simulink model "dbx_control"  (R2015a)
settings: Solver=FixedStepDiscrete  SolverMode=SingleTasking  StartTime=0.0  StopTime=20  FixedStep=T_ctrl  RelTol=1e-3
undefined symbols (not defined in the file): A_l_max_x, A_M, A_z_max, CG, epsilon, Flaps_ang_deg, g, Hover_eta_23, Hover_throtle_1, Hover_throtle_23, I_BAC, L_M, m, PID_phi_dot_Kd, PID_phi_dot_Ki, PID_phi_dot_Kp, PID_phi_Kd, PID_phi_Ki, PID_phi_Kp, PID_theta_dot_Kd, PID_theta_dot_Ki, PID_theta_dot_Kp, PID_theta_Kd, PID_theta_Ki, PID_theta_Kp, psi_f_i, psi_K_b, psi_tau, Roll_pich_sens, Servo_calib, T_ctrl, Throtle_sens, v_i0, Yaw_sens
libraries: DBX_model x29, DBX_Control_lib x15, simulink x7, DBX_Control x3
(part 1 of 2)
settings Model: ExtModeTrigDuration=5000  TunableVars=Flaps_ang_deg,PID_phi_Kd,PID_phi_Ki,PID_phi_Kp,PID_phi_dot_Kd,PID_phi_dot_Ki,PID_phi_dot_Kp,PID_theta_Kd,PID_theta_Ki,PID_theta_Kp,PID_theta_dot_Kd,PID_theta_dot_Ki,PID_theta_dot_Kp,Roll_pich_sens,Throtle_sens,Yaw_sens,p_K_b,p_tau,phi_K_b,phi_f_i,phi_tau,psi_K_b,psi_f_i,psi_tau,q_K_b,q_tau,r_K_b,r_tau,theta_K_b,theta_f_i,theta_tau  TunableVarsStorageClass=Auto,Auto,Auto,Auto,Auto,Auto,Auto,Auto,Auto,Auto,Auto,Auto,Auto,Auto,Auto,Auto,Auto,Auto,Auto,Auto,Auto,Auto,Auto,Auto,Auto,Auto,Auto,Auto,Auto,Auto,Auto  TunableVarsTypeQualifier=,,,,,,,,,,,,,,,,,,,,,,,,,,,,,,  Creator=DavidTorres  LastModifiedBy=david
settings DataIOCC: LimitDataPoints=off  SaveOutput=off  SignalLogging=off  DSMLogging=off  VisualizeSimOutput=off  SaveTime=off
settings OptimizationCC: InlineParams=on  UseDivisionForNetSlopeComputation=on  UseFloatMulNetSlope=on  UseSpecifiedMinMax=on  InlineInvariantSignals=on  StrengthReduction=on  ZeroExternalMemoryAtStartup=off  ZeroInternalMemoryAtStartup=off  NoFixptDivByZeroProtection=on  EfficientFloat2IntCast=on  OptimizeModelRefInitCode=on  MaxStackSize=64  SimCompilerOptimization=on
settings DebuggingCC: AlgebraicLoopMsg=error  SaveWithParameterizedLinksMsg=none  IntegerOverflowMsg=error  StrictBusMsg=ErrorOnBusTreatedAsVector  IntegerSaturationMsg=error
settings HardwareCC: ProdLargestAtomicInteger=Long  ProdLargestAtomicFloat=Float  ProdIntDivRoundTo=Zero  ProdEndianess=LittleEndian  ProdHWDeviceType=ARM Compatible->ARM 7  TargetLongLongMode=on  TargetIntDivRoundTo=Zero  TargetEndianess=LittleEndian  TargetHWDeviceType=MATLAB Host  ProdEqTarget=off
settings ModelReferenceCC: ModelReferenceNumInstancesAllowed=Single  ModelReferencePassRootInputsByReference=off
settings RTWCC: SystemTargetFile=ert.tlc  GenCodeOnly=on  TemplateMakefile=ert_default_tmf  Description=Embedded Coder  BuildConfiguration=Faster Runs
settings CodeAppCC: IgnoreCustomStorageClasses=off
settings ERTTargetCC: GenerateSampleERTMain=off  ParMdlRefBuildCompliant=on  CompOptLevelCompliant=on  ConcurrentExecutionCompliant=on  CombineSignalStateStructs=on  SuppressErrorStatus=on  ERTFirstTimeCompliant=on  SupportNonFinite=off  SupportComplex=off  SupportContinuousTime=off  ModelStepFunctionPrototypeControlCompliant=on  CPPClassGenCompliant=on  InlinedParameterPlacement=Hierarchical  ERTCustomFileTemplate=example_file_process.tlc

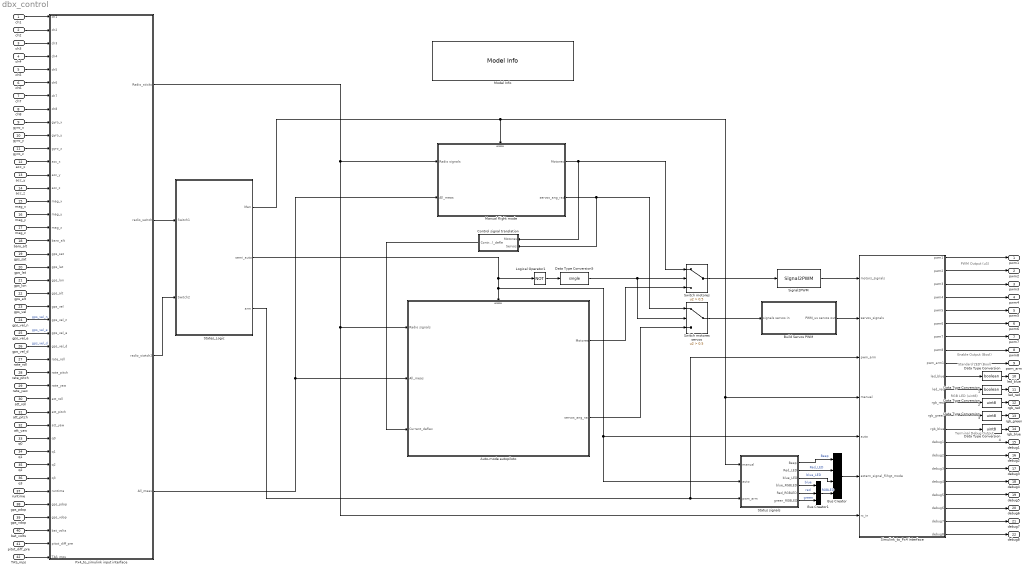
== system dbx_control ==
  note: Terminal Debug Output
  note: RGB LED (uint8)
  note: Standard LED (Bool)
  note: PWM Output (uS)
  note: Enable Output (Bool)
  ch1 : Inport  OutDataTypeStr=double  PortDimensions=[1,1]  SampleTime=T_ctrl
  ch2 : Inport  Port=2  OutDataTypeStr=double  PortDimensions=[1,1]  SampleTime=T_ctrl
  ch3 : Inport  Port=3  OutDataTypeStr=double  PortDimensions=[1,1]  SampleTime=T_ctrl
  ch4 : Inport  Port=4  OutDataTypeStr=double  PortDimensions=[1,1]  SampleTime=T_ctrl
  ch5 : Inport  Port=5  OutDataTypeStr=double  PortDimensions=[1,1]  SampleTime=T_ctrl
  ch6 : Inport  Port=6  OutDataTypeStr=double  PortDimensions=[1,1]  SampleTime=T_ctrl
  ch7 : Inport  Port=7  OutDataTypeStr=double  PortDimensions=[1,1]  SampleTime=T_ctrl
  ch8 : Inport  Port=8  OutDataTypeStr=double  PortDimensions=[1,1]  SampleTime=T_ctrl
  gyro_x : Inport  Port=9  OutDataTypeStr=double  PortDimensions=[1,1]  SampleTime=T_ctrl
  gyro_y : Inport  Port=10  OutDataTypeStr=double  PortDimensions=[1,1]  SampleTime=T_ctrl
  gyro_z : Inport  Port=11  OutDataTypeStr=double  PortDimensions=[1,1]  SampleTime=T_ctrl
  acc_x : Inport  Port=12  OutDataTypeStr=double  PortDimensions=[1,1]  SampleTime=T_ctrl
  acc_y : Inport  Port=13  OutDataTypeStr=double  PortDimensions=[1,1]  SampleTime=T_ctrl
  acc_z : Inport  Port=14  OutDataTypeStr=double  PortDimensions=[1,1]  SampleTime=T_ctrl
  mag_x : Inport  Port=15  OutDataTypeStr=double  PortDimensions=[1,1]  SampleTime=T_ctrl
  mag_y : Inport  Port=16  OutDataTypeStr=double  PortDimensions=[1,1]  SampleTime=T_ctrl
  mag_z : Inport  Port=17  OutDataTypeStr=double  PortDimensions=[1,1]  SampleTime=T_ctrl
  baro_alt : Inport  Port=18  OutDataTypeStr=double  PortDimensions=[1,1]  SampleTime=T_ctrl
  gps_sat : Inport  Port=19  OutDataTypeStr=double  PortDimensions=[1,1]  SampleTime=T_ctrl
  gps_lat : Inport  Port=20  OutDataTypeStr=double  PortDimensions=[1,1]  SampleTime=T_ctrl
  gps_lon : Inport  Port=21  OutDataTypeStr=double  PortDimensions=[1,1]  SampleTime=T_ctrl
  gps_alt : Inport  Port=22  OutDataTypeStr=double  PortDimensions=[1,1]  SampleTime=T_ctrl
  gps_vel : Inport  Port=23  OutDataTypeStr=double  PortDimensions=[1,1]  SampleTime=T_ctrl
  gps_vel_n : Inport  Port=24  OutDataTypeStr=double  PortDimensions=[1,1]  SampleTime=T_ctrl
  gps_vel_e : Inport  Port=25  OutDataTypeStr=double  PortDimensions=[1,1]  SampleTime=T_ctrl
  gps_vel_d : Inport  Port=26  OutDataTypeStr=double  PortDimensions=[1,1]  SampleTime=T_ctrl
  rate_roll : Inport  Port=27  OutDataTypeStr=double  PortDimensions=[1,1]  SampleTime=T_ctrl
  rate_pitch : Inport  Port=28  OutDataTypeStr=double  PortDimensions=[1,1]  SampleTime=T_ctrl
  rate_yaw : Inport  Port=29  OutDataTypeStr=double  PortDimensions=[1,1]  SampleTime=T_ctrl
  att_roll : Inport  Port=30  OutDataTypeStr=double  PortDimensions=[1,1]  SampleTime=T_ctrl
  att_pitch : Inport  Port=31  OutDataTypeStr=double  PortDimensions=[1,1]  SampleTime=T_ctrl
  att_yaw : Inport  Port=32  OutDataTypeStr=double  PortDimensions=[1,1]  SampleTime=T_ctrl
  q0 : Inport  Port=33  OutDataTypeStr=double  PortDimensions=[1,1]  SampleTime=T_ctrl
  q1 : Inport  Port=34  OutDataTypeStr=double  PortDimensions=[1,1]  SampleTime=T_ctrl
  q2 : Inport  Port=35  OutDataTypeStr=double  PortDimensions=[1,1]  SampleTime=T_ctrl
  q3 : Inport  Port=36  OutDataTypeStr=double  PortDimensions=[1,1]  SampleTime=T_ctrl
  runtime : Inport  Port=37  OutDataTypeStr=double  PortDimensions=[1,1]  SampleTime=T_ctrl
  gps_pdop : Inport  Port=38  OutDataTypeStr=double  PortDimensions=[1,1]  SampleTime=T_ctrl
  gps_vdop : Inport  Port=39  OutDataTypeStr=double  PortDimensions=[1,1]  SampleTime=T_ctrl
  bat_volts : Inport  Port=40  OutDataTypeStr=double  PortDimensions=[1,1]  SampleTime=T_ctrl
  pitot_diff_pre : Inport  Port=41  OutDataTypeStr=double  SampleTime=T_ctrl
  TAS_mps : Inport  Port=42  OutDataTypeStr=double  SampleTime=T_ctrl
  Auto-mode autopiloto : Subsystem  TreatAsAtomicUnit=on
  Build Servos PWM : Subsystem  TreatAsAtomicUnit=on
  Bus Creator : BusCreator
  Bus Creator1 : BusCreator  Inputs=3
  Control signal translation : Subsystem  TreatAsAtomicUnit=on
  Data Type Conversion : DataTypeConversion  OutDataTypeStr=boolean
  Data Type Conversion1 : DataTypeConversion  OutDataTypeStr=boolean
  Data Type Conversion2 : DataTypeConversion  OutDataTypeStr=uint8
  Data Type Conversion3 : DataTypeConversion  OutDataTypeStr=uint8
  Data Type Conversion4 : DataTypeConversion  OutDataTypeStr=uint8
  Data Type Conversion5 : DataTypeConversion  OutDataTypeStr=single
  Logical Operator1 : Logic  Operator=NOT  IconShape=distinctive  AllPortsSameDT=off  OutDataTypeStr=boolean
  Manual flight mode : Subsystem  TreatAsAtomicUnit=on
  Model Info : simulink/Model-Wide Utilities/Model Info  Frame=on  DisplayStringWithTags=|  HorizontalTextAlignment=Center  LeftAlignmentValue=0.5  SourceBlockDiagram=dbx_control  TagMaxNumber=20
      | Model Info
      | 
      | Creado por %<Creator>
      | Modificado el %<LastModificationDate> por %<LastModifiedBy>
      | Version %<ModelVersion>
  Px4_to_simulink input interface : Subsystem
  Signal2PWM : DBX_model/Signal2PWM  b=1  d=0  a=DBX_PWM.Motors.Max_PWM  c=DBX_PWM.Motors.Min_PWM
  Simulink_to_Px4 interface : Subsystem
  States_Logic : Subsystem
  Status signals : Subsystem  TreatAsAtomicUnit=on
  Switch motores : Switch  Criteria=u2 > Threshold  Threshold=0.5
  Switch motores servos : Switch  Criteria=u2 > Threshold  Threshold=0.5
  pwm1 : Outport  PortDimensions=[1,1]
  pwm2 : Outport  Port=2  PortDimensions=[1,1]
  pwm3 : Outport  Port=3  PortDimensions=[1,1]
  pwm4 : Outport  Port=4  PortDimensions=[1,1]
  pwm5 : Outport  Port=5  PortDimensions=[1,1]
  pwm6 : Outport  Port=6  PortDimensions=[1,1]
  pwm7 : Outport  Port=7  PortDimensions=[1,1]
  pwm8 : Outport  Port=8  PortDimensions=[1,1]
  pwm_arm : Outport  Port=9  PortDimensions=[1,1]
  led_blue : Outport  Port=10  OutDataTypeStr=boolean  PortDimensions=[1,1]
  led_red : Outport  Port=11  OutDataTypeStr=boolean  PortDimensions=[1,1]
  rgb_red : Outport  Port=12  OutDataTypeStr=uint8  PortDimensions=[1,1]
  rgb_green : Outport  Port=13  OutDataTypeStr=uint8  PortDimensions=[1,1]
  rgb_blue : Outport  Port=14  OutDataTypeStr=uint8  PortDimensions=[1,1]
  debug1 : Outport  Port=15  PortDimensions=[1,1]
  debug2 : Outport  Port=16  PortDimensions=[1,1]
  debug3 : Outport  Port=17  PortDimensions=[1,1]
  debug4 : Outport  Port=18  PortDimensions=[1,1]
  debug5 : Outport  Port=19  PortDimensions=[1,1]
  debug6 : Outport  Port=20  PortDimensions=[1,1]
  debug7 : Outport  Port=21  PortDimensions=[1,1]
  debug8 : Outport  Port=22  PortDimensions=[1,1]
  wires:
  Switch motores/1 -> Signal2PWM/1
  Switch motores servos/1 -> Build Servos PWM/1(signals servos in)
  Status signals/1(Beep) -> Bus Creator/1  "Beep"
  Status signals/2(Red_LED) -> Bus Creator/2  "Red_LED"
  Status signals/3(blue_LED) -> Bus Creator/3  "blue_LED"
  Status signals/4(blue_RGBLED) -> Bus Creator1/1  "blue"
  Status signals/5(Red_RGBLED) -> Bus Creator1/2  "red"
  Status signals/6(green_RGBLED) -> Bus Creator1/3  "green"
  Bus Creator1/1 -> Bus Creator/4  "RGBLED"
  Simulink_to_Px4 interface/1(pwm1) -> pwm1/1
  Simulink_to_Px4 interface/2(pwm2) -> pwm2/1
  Simulink_to_Px4 interface/3(pwm3) -> pwm3/1
  Simulink_to_Px4 interface/4(pwm4) -> pwm4/1
  Simulink_to_Px4 interface/5(pwm5) -> pwm5/1
  Simulink_to_Px4 interface/6(pwm6) -> pwm6/1
  Simulink_to_Px4 interface/7(pwm7) -> pwm7/1
  Simulink_to_Px4 interface/8(pwm8) -> pwm8/1
  Simulink_to_Px4 interface/10(led_blue) -> Data Type Conversion/1
  Simulink_to_Px4 interface/11(led_red) -> Data Type Conversion1/1
  Simulink_to_Px4 interface/15(debug1) -> debug1/1
  Simulink_to_Px4 interface/17(debug3) -> debug3/1
  Simulink_to_Px4 interface/18(debug4) -> debug4/1
  Simulink_to_Px4 interface/9(pwm_arm1) -> pwm_arm/1
  Simulink_to_Px4 interface/12(rgb_red) -> Data Type Conversion2/1
  Simulink_to_Px4 interface/13(rgb_green) -> Data Type Conversion3/1
  Simulink_to_Px4 interface/14(rgb_blue) -> Data Type Conversion4/1
  Simulink_to_Px4 interface/20(debug6) -> debug6/1
  Simulink_to_Px4 interface/21(debug7) -> debug7/1
  Simulink_to_Px4 interface/22(debug8) -> debug8/1
  Simulink_to_Px4 interface/19(debug5) -> debug5/1
  Data Type Conversion/1 -> led_blue/1
  Data Type Conversion1/1 -> led_red/1
  Data Type Conversion2/1 -> rgb_red/1
  Data Type Conversion3/1 -> rgb_green/1
  Data Type Conversion4/1 -> rgb_blue/1
  Simulink_to_Px4 interface/16(debug2) -> debug2/1
  Signal2PWM/1 -> Simulink_to_Px4 interface/1(motors_signals)
  Build Servos PWM/1(PWM_us servos out) -> Simulink_to_Px4 interface/2(servos_signals)
  Bus Creator/1 -> Simulink_to_Px4 interface/6(extern_signal_flihgt_mode)
  Manual flight mode/2(servos_ang_rad) -> Switch motores servos/1, Control signal translation/2(Servos)
  Auto-mode autopiloto/1(Motores) -> Switch motores/3
  Auto-mode autopiloto/2(servos_ang_rad) -> Switch motores servos/3
  Data Type Conversion5/1 -> Switch motores/2, Switch motores servos/2
  Px4_to_simulink input interface/4(All_meas) -> Auto-mode autopiloto/2(All_meas), Manual flight mode/2(All_meas)
  Px4_to_simulink input interface/1(Radio_sticks) -> Manual flight mode/1(Radio signals), Simulink_to_Px4 interface/7(rc_in), Auto-mode autopiloto/1(Radio signals)
  Manual flight mode/1(Motores) -> Switch motores/1, Control signal translation/1(Motores)
  Control signal translation/1(Control_defle) -> Auto-mode autopiloto/3(Current_deflex)
  ch1/1 -> Px4_to_simulink input interface/1(ch1)
  ch2/1 -> Px4_to_simulink input interface/2(ch2)
  ch3/1 -> Px4_to_simulink input interface/3(ch3)
  ch4/1 -> Px4_to_simulink input interface/4(ch4)
  ch5/1 -> Px4_to_simulink input interface/5(ch5)
  ch6/1 -> Px4_to_simulink input interface/6(ch6)
  ch7/1 -> Px4_to_simulink input interface/7(ch7)
  ch8/1 -> Px4_to_simulink input interface/8(ch8)
  gyro_x/1 -> Px4_to_simulink input interface/9(gyro_x)
  gyro_y/1 -> Px4_to_simulink input interface/10(gyro_y)
  gyro_z/1 -> Px4_to_simulink input interface/11(gyro_z)
  acc_x/1 -> Px4_to_simulink input interface/12(acc_x)
  acc_y/1 -> Px4_to_simulink input interface/13(acc_y)
  acc_z/1 -> Px4_to_simulink input interface/14(acc_z)
  mag_z/1 -> Px4_to_simulink input interface/17(mag_z)
  mag_y/1 -> Px4_to_simulink input interface/16(mag_y)
  mag_x/1 -> Px4_to_simulink input interface/15(mag_x)
  baro_alt/1 -> Px4_to_simulink input interface/18(baro_alt)
  gps_sat/1 -> Px4_to_simulink input interface/19(gps_sat)
  gps_lat/1 -> Px4_to_simulink input interface/20(gps_lat)
  gps_lon/1 -> Px4_to_simulink input interface/21(gps_lon)
  gps_alt/1 -> Px4_to_simulink input interface/22(gps_alt)
  gps_vel/1 -> Px4_to_simulink input interface/23(gps_vel)
  gps_vel_e/1 -> Px4_to_simulink input interface/25(gps_vel_e)  "gps_vel_e"
  gps_vel_n/1 -> Px4_to_simulink input interface/24(gps_vel_n)  "gps_vel_n"
  gps_vel_d/1 -> Px4_to_simulink input interface/26(gps_vel_d)  "gps_vel_d"
  rate_roll/1 -> Px4_to_simulink input interface/27(rate_roll)
  rate_pitch/1 -> Px4_to_simulink input interface/28(rate_pitch)
  rate_yaw/1 -> Px4_to_simulink input interface/29(rate_yaw)
  att_roll/1 -> Px4_to_simulink input interface/30(att_roll)
  att_pitch/1 -> Px4_to_simulink input interface/31(att_pitch)
  att_yaw/1 -> Px4_to_simulink input interface/32(att_yaw)
  q0/1 -> Px4_to_simulink input interface/33(q0)
  q1/1 -> Px4_to_simulink input interface/34(q1)
  q2/1 -> Px4_to_simulink input interface/35(q2)
  q3/1 -> Px4_to_simulink input interface/36(q3)
  runtime/1 -> Px4_to_simulink input interface/37(runtime)
  gps_pdop/1 -> Px4_to_simulink input interface/38(gps_pdop)
  gps_vdop/1 -> Px4_to_simulink input interface/39(gps_vdop)
  bat_volts/1 -> Px4_to_simulink input interface/40(bat_volts)
  pitot_diff_pre/1 -> Px4_to_simulink input interface/41(pitot_diff_pre)
  TAS_mps/1 -> Px4_to_simulink input interface/42(TAS_mps)
  States_Logic/3(arm) -> Simulink_to_Px4 interface/3(pwm_arm), Status signals/3(pwm_arm)
  States_Logic/1(Man) -> Manual flight mode/Enable, Simulink_to_Px4 interface/4(manual), Status signals/1(manual)
  States_Logic/2(semi_auto) -> Logical Operator1/1, Simulink_to_Px4 interface/5(auto), Status signals/2(auto), Auto-mode autopiloto/Enable
  Px4_to_simulink input interface/3(radio_siwtch2) -> States_Logic/2(Switch2)
  Logical Operator1/1 -> Data Type Conversion5/1
  Px4_to_simulink input interface/2(radio_switch) -> States_Logic/1(Switch1)

== system dbx_control/Auto-mode autopiloto ==
  Radio signals : Inport
  All_meas : Inport  Port=2
  Current_deflex : Inport  Port=3
  Enable : EnablePort  ShowOutputPort=on
  Activation bus : Subsystem  TreatAsAtomicUnit=on
  DBX advance control system : Subsystem
  Demux : Demux  Outputs=7
  "Ground " : Ground
  Initial conditions : Subsystem  TreatAsAtomicUnit=on
  Mux : Mux  Inputs=3
  Mux1 : Mux  Inputs=7
  Saturation : Saturate  UpperLimit=1  LowerLimit=0
  Saturation1 : Saturate  UpperLimit=deg2rad(90)  LowerLimit=-deg2rad(90)
  Sensibilidades Radio : Subsystem  TreatAsAtomicUnit=on
  Sup2Servo Lin conversion : DBX_model/Sup2Servo Lin conversion  Gain=Servo_calib.Servo1.Pendiente_Sup_Servo  Bias=Servo_calib.Servo1.Sup_rad_0
  Sup2Servo Lin conversion1 : DBX_model/Sup2Servo Lin conversion  Gain=Servo_calib.Servo2.Pendiente_Sup_Servo  Bias=Servo_calib.Servo2.Sup_rad_0
  Sup2Servo Lin conversion2 : DBX_model/Sup2Servo Lin conversion  Gain=Servo_calib.Servo3.Pendiente_Sup_Servo  Bias=Servo_calib.Servo3.Sup_rad_0
  Sup2Servo Lin conversion3 : DBX_model/Sup2Servo Lin conversion  Gain=Servo_calib.Servo4.Pendiente_Sup_Servo  Bias=Servo_calib.Servo4.Sup_rad_0
  Sup2Servo Lin conversion4 : DBX_model/Sup2Servo Lin conversion  Gain=Servo_calib.Servo5.Pendiente_Sup_Servo  Bias=Servo_calib.Servo5.Sup_rad_0
  Sup2Servo Lin conversion5 : DBX_model/Sup2Servo Lin conversion  Gain=Servo_calib.Servo6.Pendiente_Sup_Servo  Bias=Servo_calib.Servo6.Sup_rad_0
  Sup2Servo Lin conversion6 : DBX_model/Sup2Servo Lin conversion  Gain=Servo_calib.Servo7.Pendiente_Sup_Servo  Bias=Servo_calib.Servo7.Sup_rad_0
  Terminator : Terminator
  Motores : Outport
  servos_ang_rad : Outport  Port=2
  wires:
  DBX advance control system/1(Mot_throtles) -> Saturation/1
  Saturation/1 -> Motores/1
  Mux1/1 -> Saturation1/1
  Saturation1/1 -> servos_ang_rad/1
  Sup2Servo Lin conversion/1 -> Mux1/1
  Sup2Servo Lin conversion1/1 -> Mux1/2
  Sup2Servo Lin conversion2/1 -> Mux1/3
  Sup2Servo Lin conversion3/1 -> Mux1/4
  Sup2Servo Lin conversion4/1 -> Mux1/5
  Sup2Servo Lin conversion5/1 -> Mux1/6
  Sup2Servo Lin conversion6/1 -> Mux1/7
  All_meas/1 -> Initial conditions/1(All_meas), DBX advance control system/5(All_meas)
  DBX advance control system/3(surf_angles) -> Demux/1
  Demux/1 -> Sup2Servo Lin conversion/1
  Demux/2 -> Sup2Servo Lin conversion1/1
  Demux/3 -> Sup2Servo Lin conversion2/1
  Demux/4 -> Sup2Servo Lin conversion3/1
  Demux/5 -> Sup2Servo Lin conversion4/1
  Demux/6 -> Sup2Servo Lin conversion5/1
  Demux/7 -> Sup2Servo Lin conversion6/1
  Radio signals/1 -> Sensibilidades Radio/1(Radio_in)
  Sensibilidades Radio/1(Acc_z_mps2) -> DBX advance control system/2(Acc_z(mps2))
  Mux/1 -> DBX advance control system/3(Att_ref(rad))
  "Ground "/1 -> DBX advance control system/1(Vel_ref_yaw(mps))
  Sensibilidades Radio/2(Roll(rad)) -> Mux/1
  Sensibilidades Radio/4(Yaw(radps)) -> DBX advance control system/4(Yaw_rate_ref(rad)), Mux/3
  Sensibilidades Radio/3(Pitch(rad)) -> Mux/2
  Activation bus/1(Activation bus) -> DBX advance control system/8(activation_bus)
  Enable/1 -> DBX advance control system/9(Int_reset), Activation bus/2(Activation), Activation bus/1(Activation1)
  Initial conditions/1(Init_cond) -> DBX advance control system/6(Init_cond)
  Current_deflex/1 -> DBX advance control system/7(Init_deflect)
  DBX advance control system/2(Control_signals) -> Terminator/1

== system dbx_control/Build Servos PWM ==
  signals servos in : Inport
  Demux : Demux  Outputs=7
  Mux : Mux  Inputs=7
  Signal2PWM{,1..6} (7 alike) : DBX_model/Signal2PWM  b=deg2rad(90)  d=-deg2rad(90)  a=DBX_PWM.Servos.Max_PWM  c=DBX_PWM.Servos.Min_PWM
  PWM_us servos out : Outport
  wires:
  Mux/1 -> PWM_us servos out/1
  signals servos in/1 -> Demux/1
  Demux/6 -> Signal2PWM5/1
  Demux/5 -> Signal2PWM4/1
  Demux/4 -> Signal2PWM3/1
  Demux/3 -> Signal2PWM2/1
  Demux/2 -> Signal2PWM1/1
  Demux/1 -> Signal2PWM/1
  Signal2PWM/1 -> Mux/1
  Signal2PWM1/1 -> Mux/2
  Signal2PWM3/1 -> Mux/4
  Signal2PWM4/1 -> Mux/5
  Signal2PWM2/1 -> Mux/3
  Signal2PWM5/1 -> Mux/6
  Demux/7 -> Signal2PWM6/1
  Signal2PWM6/1 -> Mux/7

== system dbx_control/Control signal translation ==
  Motores : Inport
  Servos : Inport  Port=2
  Demux : Demux  Outputs=3
  Ground{,1..4} (5 alike) : Ground
  Mux1 : Mux  Inputs=9
  Selector : Selector  InputPortWidth=7  Indices=3
  Servo2Sup Lin conversion : DBX_model/Servo2Sup Lin conversion  Gain=Servo_calib.Servo3.Pendiente_Sup_Servo  Bias=Servo_calib.Servo3.Sup_rad_0
  Control_defle : Outport
  wires:
  Mux1/1 -> Control_defle/1
  Demux/1 -> Mux1/1
  Servos/1 -> Selector/1
  Demux/2 -> Mux1/3
  Demux/3 -> Mux1/5
  Ground/1 -> Mux1/2
  Ground1/1 -> Mux1/4
  Ground2/1 -> Mux1/7
  Ground3/1 -> Mux1/8
  Ground4/1 -> Mux1/9
  Servo2Sup Lin conversion/1 -> Mux1/6
  Motores/1 -> Demux/1
  Selector/1 -> Servo2Sup Lin conversion/1

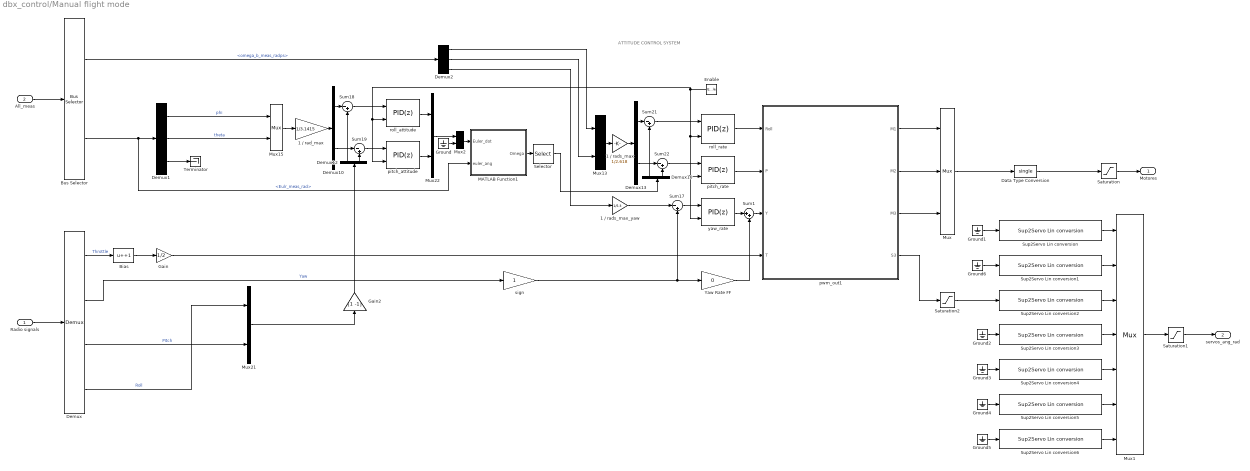
== system dbx_control/Manual flight mode ==
  note: ATTITUDE CONTROL SYSTEM
  Radio signals : Inport
  All_meas : Inport  Port=2
  Enable : EnablePort  ShowOutputPort=on
  1 / rad_max : Gain  Gain=1/3.1415
  1 / rads_max : Gain  Gain=1/2.618
  1 / rads_max_yaw : Gain  Gain=1/5.3
  Bias : Bias  Bias=+1
  Bus Selector : BusSelector  OutputSignals=Meas.omega_b_meas_radps,Meas.Eulr_meas_rad
  Data Type Conversion : DataTypeConversion  OutDataTypeStr=single
  Demux : Demux
  Demux1 : Demux  Outputs=3
  Demux{10,12..13,16} (4 alike) : Demux  Outputs=2
  Demux2 : Demux  Outputs=3
  Gain : Gain  Gain=1/2
  Gain2 : Gain  Gain=[1 -1]
  Ground{,1..6} (7 alike) : Ground
  MATLAB Function1 : MATLAB Function  TreatAsAtomicUnit=on
  Mux : Mux  Inputs=3
  Mux1 : Mux  Inputs=7
  Mux{13,15,21..22} (4 alike) : Mux  Inputs=2
  Mux2 : Mux  Inputs=[2,1]
  Saturation : Saturate  UpperLimit=1  LowerLimit=0
  Saturation1 : Saturate  UpperLimit=deg2rad(90)  LowerLimit=-deg2rad(90)  OutDataTypeStr=single
  Saturation2 : Saturate  UpperLimit=deg2rad(20)  LowerLimit=-deg2rad(20)
  Selector : Selector  InputPortWidth=3  Indices=[1:2]
  Sum1 : Sum  Inputs=|++
  Sum{17..19,21..22} (5 alike) : Sum  Inputs=|-+
  Sup2Servo Lin conversion : DBX_model/Sup2Servo Lin conversion  Gain=Servo_calib.Servo1.Pendiente_Sup_Servo  Bias=Servo_calib.Servo1.Sup_rad_0
  Sup2Servo Lin conversion1 : DBX_model/Sup2Servo Lin conversion  Gain=Servo_calib.Servo2.Pendiente_Sup_Servo  Bias=Servo_calib.Servo2.Sup_rad_0
  Sup2Servo Lin conversion2 : DBX_model/Sup2Servo Lin conversion  Gain=Servo_calib.Servo3.Pendiente_Sup_Servo  Bias=Servo_calib.Servo3.Sup_rad_0
  Sup2Servo Lin conversion3 : DBX_model/Sup2Servo Lin conversion  Gain=Servo_calib.Servo4.Pendiente_Sup_Servo  Bias=Servo_calib.Servo4.Sup_rad_0
  Sup2Servo Lin conversion4 : DBX_model/Sup2Servo Lin conversion  Gain=Servo_calib.Servo5.Pendiente_Sup_Servo  Bias=Servo_calib.Servo5.Sup_rad_0
  Sup2Servo Lin conversion5 : DBX_model/Sup2Servo Lin conversion  Gain=Servo_calib.Servo6.Pendiente_Sup_Servo  Bias=Servo_calib.Servo6.Sup_rad_0
  Sup2Servo Lin conversion6 : DBX_model/Sup2Servo Lin conversion  Gain=Servo_calib.Servo7.Pendiente_Sup_Servo  Bias=Servo_calib.Servo7.Sup_rad_0
  Terminator : Terminator
  Yaw Rate FF : Gain  Gain=0
  pitch_attitude : simulink/Continuous/PID Controller  Controller=PID  TimeDomain=Discrete-time  SampleTime=-1  IntegratorMethod=Forward Euler  FilterMethod=Forward Euler  Form=Parallel  UseFilter=on  ControllerParametersSource=internal  P=PID_theta_Kp  I=PID_theta_Ki  D=PID_theta_Kd  N=100  InitialConditionSource=internal  InitialConditionForIntegrator=0  InitialConditionForFilter=0  ExternalReset=either  LimitOutput=on  UpperSaturationLimit=1  LowerSaturationLimit=-1  LinearizeAsGain=on  AntiWindupMode=none  Kb=1  TrackingMode=off  Kt=1  PParamMin=[]  PParamMax=[]  IParamMin=[]  IParamMax=[]  DParamMin=[]  DParamMax=[]  NParamMin=[]  NParamMax=[]  KbParamMin=[]  KbParamMax=[]  KtParamMin=[]  KtParamMax=[]  POutMin=[]  POutMax=[]  IOutMin=[]  IOutMax=[]  DOutMin=[]  DOutMax=[]  NOutMin=[]  NOutMax=[]  KbOutMin=[]  KbOutMax=[]  KtOutMin=[]  KtOutMax=[]  IntegratorOutMin=[]  IntegratorOutMax=[]  FilterOutMin=[]  FilterOutMax=[]  SumOutMin=[]  SumOutMax=[]  SumI1OutMin=[]  SumI1OutMax=[]  SumI2OutMin=[]  SumI2OutMax=[]  SumI3OutMin=[]  SumI3OutMax=[]  SumDOutMin=[]  SumDOutMax=[]  SaturationOutMin=[]  SaturationOutMax=[]  IntegratorContinuousStateAttributes=''  IntegratorStateMustResolveToSignalObject=off  IntegratorRTWStateStorageClass=Auto  FilterContinuousStateAttributes=''  FilterStateMustResolveToSignalObject=off  FilterRTWStateStorageClass=Auto  DifferentiatorICPrevScaledInput=0  DifferentiatorOutMin=[]  DifferentiatorOutMax=[]
  pitch_rate : simulink/Continuous/PID Controller  Controller=PID  TimeDomain=Discrete-time  SampleTime=-1  IntegratorMethod=Forward Euler  FilterMethod=Forward Euler  Form=Parallel  UseFilter=on  ControllerParametersSource=internal  P=PID_theta_dot_Kp  I=PID_theta_dot_Ki  D=PID_theta_dot_Kd  N=100  InitialConditionSource=internal  InitialConditionForIntegrator=0  InitialConditionForFilter=0  ExternalReset=either  LimitOutput=on  UpperSaturationLimit=1  LowerSaturationLimit=-1  LinearizeAsGain=on  AntiWindupMode=none  Kb=1  TrackingMode=off  Kt=1  PParamMin=[]  PParamMax=[]  IParamMin=[]  IParamMax=[]  DParamMin=[]  DParamMax=[]  NParamMin=[]  NParamMax=[]  KbParamMin=[]  KbParamMax=[]  KtParamMin=[]  KtParamMax=[]  POutMin=[]  POutMax=[]  IOutMin=[]  IOutMax=[]  DOutMin=[]  DOutMax=[]  NOutMin=[]  NOutMax=[]  KbOutMin=[]  KbOutMax=[]  KtOutMin=[]  KtOutMax=[]  IntegratorOutMin=[]  IntegratorOutMax=[]  FilterOutMin=[]  FilterOutMax=[]  SumOutMin=[]  SumOutMax=[]  SumI1OutMin=[]  SumI1OutMax=[]  SumI2OutMin=[]  SumI2OutMax=[]  SumI3OutMin=[]  SumI3OutMax=[]  SumDOutMin=[]  SumDOutMax=[]  SaturationOutMin=[]  SaturationOutMax=[]  IntegratorContinuousStateAttributes=''  IntegratorStateMustResolveToSignalObject=off  IntegratorRTWStateStorageClass=Auto  FilterContinuousStateAttributes=''  FilterStateMustResolveToSignalObject=off  FilterRTWStateStorageClass=Auto  DifferentiatorICPrevScaledInput=0  DifferentiatorOutMin=[]  DifferentiatorOutMax=[]
  pwm_out1 : MATLAB Function  TreatAsAtomicUnit=on  SystemSampleTime=T_ctrl
  roll_attitude : simulink/Continuous/PID Controller  Controller=PID  TimeDomain=Discrete-time  SampleTime=-1  IntegratorMethod=Forward Euler  FilterMethod=Forward Euler  Form=Parallel  UseFilter=on  ControllerParametersSource=internal  P=PID_phi_Kp  I=PID_phi_Ki  D=PID_phi_Kd  N=100  InitialConditionSource=internal  InitialConditionForIntegrator=0  InitialConditionForFilter=0  ExternalReset=either  LimitOutput=on  UpperSaturationLimit=1  LowerSaturationLimit=-1  LinearizeAsGain=on  AntiWindupMode=none  Kb=1  TrackingMode=off  Kt=1  PParamMin=[]  PParamMax=[]  IParamMin=[]  IParamMax=[]  DParamMin=[]  DParamMax=[]  NParamMin=[]  NParamMax=[]  KbParamMin=[]  KbParamMax=[]  KtParamMin=[]  KtParamMax=[]  POutMin=[]  POutMax=[]  IOutMin=[]  IOutMax=[]  DOutMin=[]  DOutMax=[]  NOutMin=[]  NOutMax=[]  KbOutMin=[]  KbOutMax=[]  KtOutMin=[]  KtOutMax=[]  IntegratorOutMin=[]  IntegratorOutMax=[]  FilterOutMin=[]  FilterOutMax=[]  SumOutMin=[]  SumOutMax=[]  SumI1OutMin=[]  SumI1OutMax=[]  SumI2OutMin=[]  SumI2OutMax=[]  SumI3OutMin=[]  SumI3OutMax=[]  SumDOutMin=[]  SumDOutMax=[]  SaturationOutMin=[]  SaturationOutMax=[]  IntegratorContinuousStateAttributes=''  IntegratorStateMustResolveToSignalObject=off  IntegratorRTWStateStorageClass=Auto  FilterContinuousStateAttributes=''  FilterStateMustResolveToSignalObject=off  FilterRTWStateStorageClass=Auto  DifferentiatorICPrevScaledInput=0  DifferentiatorOutMin=[]  DifferentiatorOutMax=[]
  roll_rate : simulink/Continuous/PID Controller  Controller=PID  TimeDomain=Discrete-time  SampleTime=-1  IntegratorMethod=Forward Euler  FilterMethod=Forward Euler  Form=Parallel  UseFilter=on  ControllerParametersSource=internal  P=PID_phi_dot_Kp  I=PID_phi_dot_Ki  D=PID_phi_dot_Kd  N=100  InitialConditionSource=internal  InitialConditionForIntegrator=0  InitialConditionForFilter=0  ExternalReset=either  LimitOutput=on  UpperSaturationLimit=1  LowerSaturationLimit=-1  LinearizeAsGain=on  AntiWindupMode=none  Kb=1  TrackingMode=off  Kt=1  PParamMin=[]  PParamMax=[]  IParamMin=[]  IParamMax=[]  DParamMin=[]  DParamMax=[]  NParamMin=[]  NParamMax=[]  KbParamMin=[]  KbParamMax=[]  KtParamMin=[]  KtParamMax=[]  POutMin=[]  POutMax=[]  IOutMin=[]  IOutMax=[]  DOutMin=[]  DOutMax=[]  NOutMin=[]  NOutMax=[]  KbOutMin=[]  KbOutMax=[]  KtOutMin=[]  KtOutMax=[]  IntegratorOutMin=[]  IntegratorOutMax=[]  FilterOutMin=[]  FilterOutMax=[]  SumOutMin=[]  SumOutMax=[]  SumI1OutMin=[]  SumI1OutMax=[]  SumI2OutMin=[]  SumI2OutMax=[]  SumI3OutMin=[]  SumI3OutMax=[]  SumDOutMin=[]  SumDOutMax=[]  SaturationOutMin=[]  SaturationOutMax=[]  IntegratorContinuousStateAttributes=''  IntegratorStateMustResolveToSignalObject=off  IntegratorRTWStateStorageClass=Auto  FilterContinuousStateAttributes=''  FilterStateMustResolveToSignalObject=off  FilterRTWStateStorageClass=Auto  DifferentiatorICPrevScaledInput=0  DifferentiatorOutMin=[]  DifferentiatorOutMax=[]
  sign : Gain
  yaw_rate : simulink/Continuous/PID Controller  Controller=PID  TimeDomain=Discrete-time  SampleTime=-1  IntegratorMethod=Forward Euler  FilterMethod=Forward Euler  Form=Parallel  UseFilter=on  ControllerParametersSource=internal  P=2  I=0.2  D=0  N=100  InitialConditionSource=internal  InitialConditionForIntegrator=0  InitialConditionForFilter=0  ExternalReset=either  LimitOutput=on  UpperSaturationLimit=1  LowerSaturationLimit=-1  LinearizeAsGain=on  AntiWindupMode=none  Kb=1  TrackingMode=off  Kt=1  PParamMin=[]  PParamMax=[]  IParamMin=[]  IParamMax=[]  DParamMin=[]  DParamMax=[]  NParamMin=[]  NParamMax=[]  KbParamMin=[]  KbParamMax=[]  KtParamMin=[]  KtParamMax=[]  POutMin=[]  POutMax=[]  IOutMin=[]  IOutMax=[]  DOutMin=[]  DOutMax=[]  NOutMin=[]  NOutMax=[]  KbOutMin=[]  KbOutMax=[]  KtOutMin=[]  KtOutMax=[]  IntegratorOutMin=[]  IntegratorOutMax=[]  FilterOutMin=[]  FilterOutMax=[]  SumOutMin=[]  SumOutMax=[]  SumI1OutMin=[]  SumI1OutMax=[]  SumI2OutMin=[]  SumI2OutMax=[]  SumI3OutMin=[]  SumI3OutMax=[]  SumDOutMin=[]  SumDOutMax=[]  SaturationOutMin=[]  SaturationOutMax=[]  IntegratorContinuousStateAttributes=''  IntegratorStateMustResolveToSignalObject=off  IntegratorRTWStateStorageClass=Auto  FilterContinuousStateAttributes=''  FilterStateMustResolveToSignalObject=off  FilterRTWStateStorageClass=Auto  DifferentiatorICPrevScaledInput=0  DifferentiatorOutMin=[]  DifferentiatorOutMax=[]
  Motores : Outport
  servos_ang_rad : Outport  Port=2
  wires:
  Radio signals/1 -> Demux/1
  Mux/1 -> Data Type Conversion/1
  Saturation/1 -> Motores/1
  Demux/1 -> Bias/1  "Throttle"
  Bias/1 -> Gain/1
  Demux/2 -> sign/1  "Yaw"
  Demux/3 -> Mux21/2  "Pitch"
  Demux/4 -> Mux21/1  "Roll"
  Mux1/1 -> Saturation1/1
  Saturation1/1 -> servos_ang_rad/1
  Sup2Servo Lin conversion/1 -> Mux1/1
  Sup2Servo Lin conversion1/1 -> Mux1/2
  Sup2Servo Lin conversion2/1 -> Mux1/3
  Sup2Servo Lin conversion3/1 -> Mux1/4
  Sup2Servo Lin conversion4/1 -> Mux1/5
  Sup2Servo Lin conversion5/1 -> Mux1/6
  Sup2Servo Lin conversion6/1 -> Mux1/7
  Sum21/1 -> roll_rate/1
  1 / rads_max/1 -> Demux13/1
  Demux13/2 -> Sum22/1
  Demux13/1 -> Sum21/1
  Sum17/1 -> yaw_rate/1
  Sum22/1 -> pitch_rate/1
  Mux13/1 -> 1 / rads_max/1
  pitch_rate/1 -> pwm_out1/2(P)
  Sum18/1 -> roll_attitude/1
  1 / rad_max/1 -> Demux10/1
  Demux10/2 -> Sum19/1
  Demux10/1 -> Sum18/1
  Demux2/1 -> Mux13/1
  Demux12/2 -> Sum19/2
  Demux12/1 -> Sum18/2
  Demux16/2 -> Sum22/2
  Demux16/1 -> Sum21/2
  roll_attitude/1 -> Mux22/1
  pitch_attitude/1 -> Mux22/2
  Demux2/3 -> 1 / rads_max_yaw/1
  Demux2/2 -> Mux13/2
  Sum19/1 -> pitch_attitude/1
  roll_rate/1 -> pwm_out1/1(Roll)
  1 / rads_max_yaw/1 -> Sum17/1
  Mux21/1 -> Gain2/1
  Demux1/2 -> Mux15/2  "theta"
  Mux15/1 -> 1 / rad_max/1
  Demux1/1 -> Mux15/1  "phi"
  Gain2/1 -> Demux12/1
  Enable/1 -> pitch_attitude/2, roll_attitude/2, yaw_rate/2, pitch_rate/2, roll_rate/2
  Ground1/1 -> Sup2Servo Lin conversion/1
  Ground6/1 -> Sup2Servo Lin conversion1/1
  Saturation2/1 -> Sup2Servo Lin conversion2/1
  sign/1 -> Yaw Rate FF/1, Sum17/2
  All_meas/1 -> Bus Selector/1
  Bus Selector/2 -> Demux1/1, MATLAB Function1/2(euler_ang)  "<Eulr_meas_rad>"
  Bus Selector/1 -> Demux2/1  "<omega_b_meas_radps>"
  Demux1/3 -> Terminator/1
  Gain/1 -> pwm_out1/4(T)
  Data Type Conversion/1 -> Saturation/1
  Mux22/1 -> Mux2/1
  Mux2/1 -> MATLAB Function1/1(Euler_dot)
  Ground/1 -> Mux2/2
  Selector/1 -> Demux16/1
  MATLAB Function1/1(Omega) -> Selector/1
  yaw_rate/1 -> Sum1/1
  Sum1/1 -> pwm_out1/3(Y)
  Yaw Rate FF/1 -> Sum1/2
  pwm_out1/4(S3) -> Saturation2/1
  Ground2/1 -> Sup2Servo Lin conversion3/1
  Ground3/1 -> Sup2Servo Lin conversion4/1
  Ground4/1 -> Sup2Servo Lin conversion5/1
  Ground5/1 -> Sup2Servo Lin conversion6/1
  pwm_out1/1(M1) -> Mux/1
  pwm_out1/2(M2) -> Mux/2
  pwm_out1/3(M3) -> Mux/3

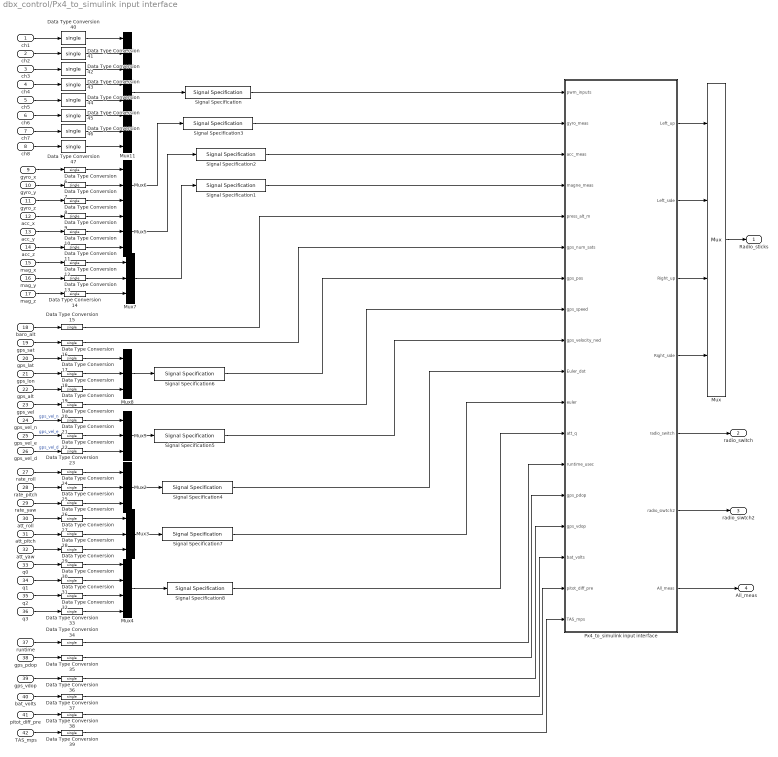
== system dbx_control/Px4_to_simulink input interface ==
  ch1 : Inport  OutDataTypeStr=double  PortDimensions=[1,1]  SampleTime=T_ctrl
  ch2 : Inport  Port=2  OutDataTypeStr=double  PortDimensions=[1,1]  SampleTime=T_ctrl
  ch3 : Inport  Port=3  OutDataTypeStr=double  PortDimensions=[1,1]  SampleTime=T_ctrl
  ch4 : Inport  Port=4  OutDataTypeStr=double  PortDimensions=[1,1]  SampleTime=T_ctrl
  ch5 : Inport  Port=5  OutDataTypeStr=double  PortDimensions=[1,1]  SampleTime=T_ctrl
  ch6 : Inport  Port=6  OutDataTypeStr=double  PortDimensions=[1,1]  SampleTime=T_ctrl
  ch7 : Inport  Port=7  OutDataTypeStr=double  PortDimensions=[1,1]  SampleTime=T_ctrl
  ch8 : Inport  Port=8  OutDataTypeStr=double  PortDimensions=[1,1]  SampleTime=T_ctrl
  gyro_x : Inport  Port=9  OutDataTypeStr=double  PortDimensions=[1,1]  SampleTime=T_ctrl
  gyro_y : Inport  Port=10  OutDataTypeStr=double  PortDimensions=[1,1]  SampleTime=T_ctrl
  gyro_z : Inport  Port=11  OutDataTypeStr=double  PortDimensions=[1,1]  SampleTime=T_ctrl
  acc_x : Inport  Port=12  OutDataTypeStr=double  PortDimensions=[1,1]  SampleTime=T_ctrl
  acc_y : Inport  Port=13  OutDataTypeStr=double  PortDimensions=[1,1]  SampleTime=T_ctrl
  acc_z : Inport  Port=14  OutDataTypeStr=double  PortDimensions=[1,1]  SampleTime=T_ctrl
  mag_x : Inport  Port=15  OutDataTypeStr=double  PortDimensions=[1,1]  SampleTime=T_ctrl
  mag_y : Inport  Port=16  OutDataTypeStr=double  PortDimensions=[1,1]  SampleTime=T_ctrl
  mag_z : Inport  Port=17  OutDataTypeStr=double  PortDimensions=[1,1]  SampleTime=T_ctrl
  baro_alt : Inport  Port=18  OutDataTypeStr=double  PortDimensions=[1,1]  SampleTime=T_ctrl
  gps_sat : Inport  Port=19  OutDataTypeStr=double  PortDimensions=[1,1]  SampleTime=T_ctrl
  gps_lat : Inport  Port=20  OutDataTypeStr=double  PortDimensions=[1,1]  SampleTime=T_ctrl
  gps_lon : Inport  Port=21  OutDataTypeStr=double  PortDimensions=[1,1]  SampleTime=T_ctrl
  gps_alt : Inport  Port=22  OutDataTypeStr=double  PortDimensions=[1,1]  SampleTime=T_ctrl
  gps_vel : Inport  Port=23  OutDataTypeStr=double  PortDimensions=[1,1]  SampleTime=T_ctrl
  gps_vel_n : Inport  Port=24  OutDataTypeStr=double  PortDimensions=[1,1]  SampleTime=T_ctrl
  gps_vel_e : Inport  Port=25  OutDataTypeStr=double  PortDimensions=[1,1]  SampleTime=T_ctrl
  gps_vel_d : Inport  Port=26  OutDataTypeStr=double  PortDimensions=[1,1]  SampleTime=T_ctrl
  rate_roll : Inport  Port=27  OutDataTypeStr=double  PortDimensions=[1,1]  SampleTime=T_ctrl
  rate_pitch : Inport  Port=28  OutDataTypeStr=double  PortDimensions=[1,1]  SampleTime=T_ctrl
  rate_yaw : Inport  Port=29  OutDataTypeStr=double  PortDimensions=[1,1]  SampleTime=T_ctrl
  att_roll : Inport  Port=30  OutDataTypeStr=double  PortDimensions=[1,1]  SampleTime=T_ctrl
  att_pitch : Inport  Port=31  OutDataTypeStr=double  PortDimensions=[1,1]  SampleTime=T_ctrl
  att_yaw : Inport  Port=32  OutDataTypeStr=double  PortDimensions=[1,1]  SampleTime=T_ctrl
  q0 : Inport  Port=33  OutDataTypeStr=double  PortDimensions=[1,1]  SampleTime=T_ctrl
  q1 : Inport  Port=34  OutDataTypeStr=double  PortDimensions=[1,1]  SampleTime=T_ctrl
  q2 : Inport  Port=35  OutDataTypeStr=double  PortDimensions=[1,1]  SampleTime=T_ctrl
  q3 : Inport  Port=36  OutDataTypeStr=double  PortDimensions=[1,1]  SampleTime=T_ctrl
  runtime : Inport  Port=37  OutDataTypeStr=double  PortDimensions=[1,1]  SampleTime=T_ctrl
  gps_pdop : Inport  Port=38  OutDataTypeStr=double  PortDimensions=[1,1]  SampleTime=T_ctrl
  gps_vdop : Inport  Port=39  OutDataTypeStr=double  PortDimensions=[1,1]  SampleTime=T_ctrl
  bat_volts : Inport  Port=40  OutDataTypeStr=double  PortDimensions=[1,1]  SampleTime=T_ctrl
  pitot_diff_pre : Inport  Port=41  OutDataTypeStr=double  SampleTime=T_ctrl
  TAS_mps : Inport  Port=42  OutDataTypeStr=double  SampleTime=T_ctrl
  Data Type Conversion{6..47} (42 alike) : DataTypeConversion  OutDataTypeStr=single
  Mux : Mux
  Mux11 : Mux  Inputs=8
  Mux{2..3,5..9} (7 alike) : Mux  Inputs=3
  Mux4 : Mux
  Px4_to_simulink input interface : Subsystem
  Signal Specification : SignalSpecification  OutDataTypeStr=single  Dimensions=[8,1]
  Signal Specification{1..7} (7 alike) : SignalSpecification  OutDataTypeStr=single  Dimensions=[3,1]
  Signal Specification8 : SignalSpecification  OutDataTypeStr=single  Dimensions=[4,1]
  Radio_sticks : Outport
  radio_switch : Outport  Port=2
  radio_siwtch2 : Outport  Port=3
  All_meas : Outport  Port=4
  wires:
  baro_alt/1 -> Data Type Conversion15/1
  gyro_z/1 -> Data Type Conversion8/1
  gyro_y/1 -> Data Type Conversion7/1
  gyro_x/1 -> Data Type Conversion6/1
  acc_z/1 -> Data Type Conversion11/1
  acc_y/1 -> Data Type Conversion10/1
  acc_x/1 -> Data Type Conversion9/1
  mag_x/1 -> Data Type Conversion12/1
  mag_y/1 -> Data Type Conversion13/1
  mag_z/1 -> Data Type Conversion14/1
  ch1/1 -> Data Type Conversion40/1
  ch2/1 -> Data Type Conversion41/1
  ch3/1 -> Data Type Conversion42/1
  ch4/1 -> Data Type Conversion43/1
  ch5/1 -> Data Type Conversion44/1
  ch6/1 -> Data Type Conversion45/1
  runtime/1 -> Data Type Conversion34/1
  ch7/1 -> Data Type Conversion46/1
  ch8/1 -> Data Type Conversion47/1
  att_roll/1 -> Data Type Conversion27/1
  att_pitch/1 -> Data Type Conversion28/1
  att_yaw/1 -> Data Type Conversion29/1
  q0/1 -> Data Type Conversion30/1
  q1/1 -> Data Type Conversion31/1
  q2/1 -> Data Type Conversion32/1
  q3/1 -> Data Type Conversion33/1
  rate_roll/1 -> Data Type Conversion24/1
  rate_pitch/1 -> Data Type Conversion25/1
  rate_yaw/1 -> Data Type Conversion26/1
  gps_vel_n/1 -> Data Type Conversion21/1  "gps_vel_n"
  gps_vel_e/1 -> Data Type Conversion22/1  "gps_vel_e"
  gps_vel_d/1 -> Data Type Conversion23/1  "gps_vel_d"
  gps_lat/1 -> Data Type Conversion17/1
  gps_lon/1 -> Data Type Conversion18/1
  gps_alt/1 -> Data Type Conversion19/1
  gps_vel/1 -> Data Type Conversion20/1
  gps_sat/1 -> Data Type Conversion16/1
  Mux2/1 -> Signal Specification4/1
  Mux3/1 -> Signal Specification7/1
  Mux4/1 -> Signal Specification8/1
  Mux5/1 -> Signal Specification2/1
  Mux6/1 -> Signal Specification3/1
  Mux8/1 -> Signal Specification6/1
  Mux7/1 -> Signal Specification1/1
  Mux11/1 -> Signal Specification/1
  Mux9/1 -> Signal Specification5/1
  gps_pdop/1 -> Data Type Conversion35/1
  gps_vdop/1 -> Data Type Conversion36/1
  bat_volts/1 -> Data Type Conversion37/1
  Signal Specification/1 -> Px4_to_simulink input interface/1(pwm_inputs)
  Signal Specification3/1 -> Px4_to_simulink input interface/2(gyro_meas)
  Signal Specification2/1 -> Px4_to_simulink input interface/3(acc_meas)
  Signal Specification1/1 -> Px4_to_simulink input interface/4(magne_meas)
  Signal Specification6/1 -> Px4_to_simulink input interface/7(gps_pos)
  Signal Specification5/1 -> Px4_to_simulink input interface/9(gps_velocity_ned)
  Signal Specification4/1 -> Px4_to_simulink input interface/10(Euler_dot)
  Signal Specification7/1 -> Px4_to_simulink input interface/11(euler)
  Signal Specification8/1 -> Px4_to_simulink input interface/12(att_q)
  pitot_diff_pre/1 -> Data Type Conversion38/1
  TAS_mps/1 -> Data Type Conversion39/1
  Data Type Conversion6/1 -> Mux6/1
  Data Type Conversion7/1 -> Mux6/2
  Data Type Conversion8/1 -> Mux6/3
  Data Type Conversion9/1 -> Mux5/1
  Data Type Conversion10/1 -> Mux5/2
  Data Type Conversion11/1 -> Mux5/3
  Data Type Conversion12/1 -> Mux7/1
  Data Type Conversion13/1 -> Mux7/2
  Data Type Conversion14/1 -> Mux7/3
  Data Type Conversion15/1 -> Px4_to_simulink input interface/5(press_alt_m)
  Data Type Conversion16/1 -> Px4_to_simulink input interface/6(gps_num_sats)
  Data Type Conversion17/1 -> Mux8/1
  Data Type Conversion18/1 -> Mux8/2
  Data Type Conversion19/1 -> Mux8/3
  Data Type Conversion20/1 -> Px4_to_simulink input interface/8(gps_speed)
  Data Type Conversion21/1 -> Mux9/1
  Data Type Conversion22/1 -> Mux9/2
  Data Type Conversion23/1 -> Mux9/3
  Data Type Conversion24/1 -> Mux2/1
  Data Type Conversion25/1 -> Mux2/2
  Data Type Conversion26/1 -> Mux2/3
  Data Type Conversion27/1 -> Mux3/1
  Data Type Conversion28/1 -> Mux3/2
  Data Type Conversion29/1 -> Mux3/3
  Data Type Conversion30/1 -> Mux4/1
  Data Type Conversion31/1 -> Mux4/2
  Data Type Conversion32/1 -> Mux4/3
  Data Type Conversion33/1 -> Mux4/4
  Data Type Conversion34/1 -> Px4_to_simulink input interface/13(runtime_usec)
  Data Type Conversion35/1 -> Px4_to_simulink input interface/14(gps_pdop)
  Data Type Conversion36/1 -> Px4_to_simulink input interface/15(gps_vdop)
  Data Type Conversion37/1 -> Px4_to_simulink input interface/16(bat_volts)
  Data Type Conversion38/1 -> Px4_to_simulink input interface/17(pitot_diff_pre)
  Data Type Conversion39/1 -> Px4_to_simulink input interface/18(TAS_mps)
  Data Type Conversion40/1 -> Mux11/1
  Data Type Conversion41/1 -> Mux11/2
  Data Type Conversion42/1 -> Mux11/3
  Data Type Conversion43/1 -> Mux11/4
  Data Type Conversion44/1 -> Mux11/5
  Data Type Conversion45/1 -> Mux11/6
  Data Type Conversion46/1 -> Mux11/7
  Data Type Conversion47/1 -> Mux11/8
  Px4_to_simulink input interface/5(radio_switch) -> radio_switch/1
  Px4_to_simulink input interface/7(All_meas) -> All_meas/1
  Px4_to_simulink input interface/6(radio_siwtch2) -> radio_siwtch2/1
  Mux/1 -> Radio_sticks/1
  Px4_to_simulink input interface/1(Left_up) -> Mux/1
  Px4_to_simulink input interface/2(Left_side) -> Mux/2
  Px4_to_simulink input interface/3(Right_up) -> Mux/3
  Px4_to_simulink input interface/4(Right_side) -> Mux/4

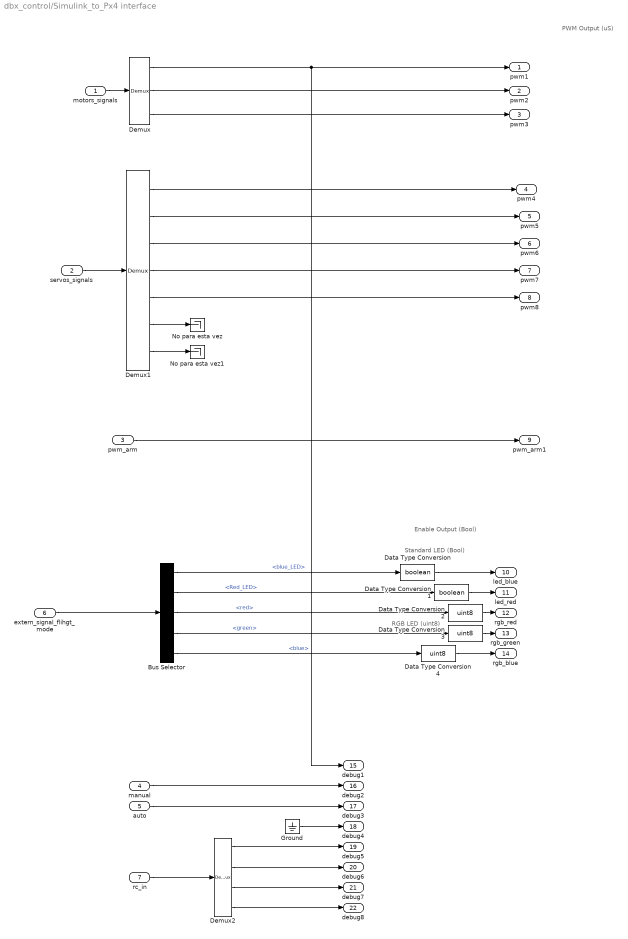
== system dbx_control/Simulink_to_Px4 interface ==
  note: RGB LED (uint8)
  note: Standard LED (Bool)
  note: PWM Output (uS)
  note: Enable Output (Bool)
  motors_signals : Inport
  servos_signals : Inport  Port=2
  pwm_arm : Inport  Port=3
  manual : Inport  Port=4
  auto : Inport  Port=5
  extern_signal_flihgt_mode : Inport  Port=6
  rc_in : Inport  Port=7
  Bus Selector : BusSelector  OutputSignals=blue_LED,Red_LED,RGBLED.red,RGBLED.green,RGBLED.blue
  Data Type Conversion : DataTypeConversion  OutDataTypeStr=boolean
  Data Type Conversion1 : DataTypeConversion  OutDataTypeStr=boolean
  Data Type Conversion2 : DataTypeConversion  OutDataTypeStr=uint8
  Data Type Conversion3 : DataTypeConversion  OutDataTypeStr=uint8
  Data Type Conversion4 : DataTypeConversion  OutDataTypeStr=uint8
  Demux : Demux  Outputs=3
  Demux1 : Demux  Outputs=7
  Demux2 : Demux
  Ground : Ground
  No para esta vez : Terminator
  No para esta vez1 : Terminator
  pwm1 : Outport  PortDimensions=1  SampleTime=T_ctrl
  pwm2 : Outport  Port=2  PortDimensions=1  SampleTime=T_ctrl
  pwm3 : Outport  Port=3  PortDimensions=1  SampleTime=T_ctrl
  pwm4 : Outport  Port=4  PortDimensions=1  SampleTime=T_ctrl
  pwm5 : Outport  Port=5  PortDimensions=1  SampleTime=T_ctrl
  pwm6 : Outport  Port=6  PortDimensions=1  SampleTime=T_ctrl
  pwm7 : Outport  Port=7  PortDimensions=1  SampleTime=T_ctrl
  pwm8 : Outport  Port=8  PortDimensions=1  SampleTime=T_ctrl
  pwm_arm1 : Outport  Port=9  PortDimensions=1  SampleTime=T_ctrl
  led_blue : Outport  Port=10  OutDataTypeStr=boolean  PortDimensions=1  SampleTime=T_ctrl
  led_red : Outport  Port=11  OutDataTypeStr=boolean  PortDimensions=1  SampleTime=T_ctrl
  rgb_red : Outport  Port=12  OutDataTypeStr=uint8  PortDimensions=1  SampleTime=T_ctrl
  rgb_green : Outport  Port=13  OutDataTypeStr=uint8  PortDimensions=1  SampleTime=T_ctrl
  rgb_blue : Outport  Port=14  OutDataTypeStr=uint8  PortDimensions=1  SampleTime=T_ctrl
  debug1 : Outport  Port=15  PortDimensions=1  SampleTime=T_ctrl
  debug2 : Outport  Port=16  PortDimensions=1  SampleTime=T_ctrl
  debug3 : Outport  Port=17  PortDimensions=1  SampleTime=T_ctrl
  debug4 : Outport  Port=18  PortDimensions=1  SampleTime=T_ctrl
  debug5 : Outport  Port=19  PortDimensions=1  SampleTime=T_ctrl
  debug6 : Outport  Port=20  PortDimensions=1  SampleTime=T_ctrl
  debug7 : Outport  Port=21  PortDimensions=1  SampleTime=T_ctrl
  debug8 : Outport  Port=22  PortDimensions=1  SampleTime=T_ctrl
  wires:
  extern_signal_flihgt_mode/1 -> Bus Selector/1
  Bus Selector/2 -> Data Type Conversion1/1  "<Red_LED>"
  pwm_arm/1 -> pwm_arm1/1
  Bus Selector/3 -> Data Type Conversion2/1  "<red>"
  Bus Selector/4 -> Data Type Conversion3/1  "<green>"
  Bus Selector/5 -> Data Type Conversion4/1  "<blue>"
  Data Type Conversion/1 -> led_blue/1
  Data Type Conversion1/1 -> led_red/1
  Data Type Conversion2/1 -> rgb_red/1
  Data Type Conversion3/1 -> rgb_green/1
  Data Type Conversion4/1 -> rgb_blue/1
  Bus Selector/1 -> Data Type Conversion/1  "<blue_LED>"
  motors_signals/1 -> Demux/1
  Demux/1 -> debug1/1, pwm1/1
  Demux/2 -> pwm2/1
  servos_signals/1 -> Demux1/1
  rc_in/1 -> Demux2/1
  manual/1 -> debug2/1
  auto/1 -> debug3/1
  Demux2/4 -> debug8/1
  Demux2/3 -> debug7/1
  Demux2/2 -> debug6/1
  Demux2/1 -> debug5/1
  Ground/1 -> debug4/1
  Demux/3 -> pwm3/1
  Demux1/1 -> pwm4/1
  Demux1/2 -> pwm5/1
  Demux1/3 -> pwm6/1
  Demux1/4 -> pwm7/1
  Demux1/5 -> pwm8/1
  Demux1/6 -> No para esta vez/1
  Demux1/7 -> No para esta vez1/1

== system dbx_control/States_Logic ==
  Switch1 : Inport
  Switch2 : Inport  Port=2
  Logical Operator1 : Logic  Operator=NOT  IconShape=distinctive  AllPortsSameDT=off  OutDataTypeStr=boolean
  Manual : Logic  IconShape=distinctive  AllPortsSameDT=off  OutDataTypeStr=boolean
  Relay : Relay  OnSwitchValue=0.6  OffSwitchValue=0.2  OutDataTypeStr=uint8
  Relay1 : Relay  OnSwitchValue=0.6  OffSwitchValue=0.2  OutDataTypeStr=uint8
  Semi_auto : Logic  IconShape=distinctive  AllPortsSameDT=off  OutDataTypeStr=boolean
  to bool : DataTypeConversion  OutDataTypeStr=boolean
  to bool1 : DataTypeConversion  OutDataTypeStr=boolean
  Man : Outport
  semi_auto : Outport  Port=2
  arm : Outport  Port=3
  wires:
  Logical Operator1/1 -> Manual/2
  Switch1/1 -> Relay/1
  Switch2/1 -> Relay1/1
  Relay/1 -> to bool/1
  Relay1/1 -> to bool1/1
  Manual/1 -> Man/1
  Semi_auto/1 -> semi_auto/1
  to bool/1 -> arm/1, Semi_auto/1, Manual/1
  to bool1/1 -> Logical Operator1/1, Semi_auto/2

== system dbx_control/Status signals ==
  manual : Inport
  auto : Inport  Port=2
  pwm_arm : Inport  Port=3
  Ground1 : Ground
  Logical Operator1 : Logic  Operator=NOT  IconShape=distinctive  AllPortsSameDT=off  OutDataTypeStr=boolean
  Beep : Outport
  Red_LED : Outport  Port=2
  blue_LED : Outport  Port=3
  blue_RGBLED : Outport  Port=4
  Red_RGBLED : Outport  Port=5
  green_RGBLED : Outport  Port=6
  wires:
  Ground1/1 -> Beep/1
  manual/1 -> Red_RGBLED/1, Red_LED/1
  auto/1 -> blue_RGBLED/1, blue_LED/1
  pwm_arm/1 -> Logical Operator1/1
  Logical Operator1/1 -> green_RGBLED/1

== system dbx_control/Auto-mode autopiloto/Activation bus ==
  Activation1 : Inport
  Activation : Inport  Port=2
  Bus Creator : BusCreator  Inputs=6
  Ground{,1..3} (4 alike) : Ground
  Activation bus : Outport
  wires:
  Ground1/1 -> Bus Creator/2  "alt_act"
  Ground2/1 -> Bus Creator/3  "vel_yaw_xy_act"
  Ground3/1 -> Bus Creator/4  "vel_yaw_z_act"
  Activation1/1 -> Bus Creator/5  "euler_act"
  Activation/1 -> Bus Creator/6  "b_rates_act"
  Bus Creator/1 -> Activation bus/1
  Ground/1 -> Bus Creator/1  "pos_xy_act"
